simulink model "different_inverter_controls_BPS"  (R2024b)
settings: Solver=ode4  StartTime=0.0  StopTime=5  FixedStep=Ts  RelTol=1e-3
InitFcn:
  | %mode_of_operation=1;
  | %BESS_control_mode=1;
  | %Gen_Q_Control =1;
  | 
  | %Exciter_init;
  | 
  | %Exciter_init
  | Xq=0.474;
  | %%====================================================
  | % ST6C Exciter Parameters
  | 
  | KPA=30;
  | KIA=59.91;
  | KFF=1;
  | KM=1;
  | KLR=22.47;
  | KCL=1.04;
  | VAMAX=7.05;
  | VAMIN=-6.11;
  | VRMAX=7.05;
  | VRMIN=-6.11;
  | ILR=5.02;
  | KG=1;
  | TG=0.024;
  | TA=0.01;
  | VBMAX=999;
  | VMMAX=7.05;
  | VMMIN=-6.11;
  | KI=0;
  | Kp=1;
  | Kc=0;
  | Vt0=0;
  | VAAMAX=VAMAX;
  | %%========================================================
  | % UEL2C parameters
  | 
  | TUQ=.005;
  | TUP=0.050;
  | TUV=0.2;
  | TQREF=0;
  | Tadj=0;
  | K1=0;
  | K2=2;
  | VBIAS=1;
  | KFB=0;
  | TUL=0;
  | VUImax=1;
  | VUImin=-1;
  | VUELmax1=1;
  | VUELmax2=1;
  | VUELmin1=-1;
  | VUELmin2=-1;
  | KUF=0;
  | KUL=0.24;
  | KUI=0.001;
  | TU1=0;TU2=0;TU3=0;TU4=0;
  | KFIX=1;
  | VF=0;
  | VFB=0;
  | %%===========================================================
  | ... (+60 lines)
values from neighbouring files (symbols this model uses):
  inv1 = struct    [multiInverterParams.m]
  kp_sync = KQ_p/10    (= 0.04)    [multiInverterParams.m]
  Vdc = 1000    [multiInverterParams.m]
  Vpp = 480    [multiInverterParams.m]
undefined symbols (not defined in the file or in its folder): D1, Delta, DiscIntNeverNeededParam, Ion, Lithium, sigbuilder_block, sps
libraries: slpidlib x34, spsThreePhaseVIMeasurementLib x31, spsThreePhaseSeriesRLCBranchLib x23, spsabctodq0Lib x22, spsPower3phInstantaneousLib x22, spsThreePhaseTransformerTwoWindingsLib x16, spsSeriesRLCBranchLib x16, spsThreePhaseSeriesRLCLoadLib x14, simulink x12, spsPLL3phLib x11, spsGroundLib x9, powerlib_extras x8
(part 2 of 9)

== system different_inverter_controls_BPS/IBR-GFM Synchro-inverter/Inverter ==
  " Reference " : Subsystem
  "            VDC1" : spsDCVoltageSourceLib/DC Voltage Source  Amplitude=Vdc  Measurements=None
  Bus Selector : BusSelector  OutputSignals=Vabc,Iabc
  DC Link : Subsystem
  From1 : From  Commented=on  GotoTag=m_batt
  From2 : From  Commented=on  GotoTag=m_inv
  Goto Tag Visibility : GotoTagVisibility  GotoTag=PLL_Freq
  Grid Inverter : Subsystem
  Inverter Control : Subsystem
  Measures : Subsystem  Commented=on
  Power Controller : Subsystem  SystemSampleTime=Ts
  Rate Transition2 : RateTransition  OutPortSampleTime=Ts_Control
  Scope : Scope
  Scope1 : Scope
  Voltage Measurement : spsVoltageMeasurementLib/Voltage Measurement  PhasorSimulation=off  OutputType=Complex  PSBequivalent=0
  A : PMIOPort  Side=Right
  B : PMIOPort  Port=2  Side=Right
  C : PMIOPort  Port=3  Side=Right
  m : Outport  VectorParamsAs1DForOutWhenUnconnected=off
  tag scope: Uref=global
  wires:
  [V_inv_mag] -> Inverter Control/5(V_inv_mag)
  [V_inv_mag] -> Power Controller/5(V_inv_mag)
  Voltage Measurement/1 -> Scope1/1
  Power Controller/2(Vdref) -> Inverter Control/4(Vdref)
  [BESS_PQf_ref] -> Power Controller/2(PQref_f)
  Rate Transition2/1 -> Bus Selector/1, Power Controller/1(m_PQ)
  Inverter Control/1(Uref) -> [Uref], Scope/1, Grid Inverter/1(Uref)
  Bus Selector/1 -> Inverter Control/1(Vabc_prim)  "<Vabc>"
  Bus Selector/2 -> Inverter Control/2(Iabc_prim)  "<Iabc>"
  Grid Inverter/1(m) -> [m_inv]
  From2/1 -> Measures/1(Grid)
  From1/1 -> Measures/2(Battery)
  Measures/1(m) -> m/1
  [m_inv] -> Rate Transition2/1
  Power Controller/1(theta) -> Inverter Control/3(theta)
  [theta_wt] -> Power Controller/3(Input)
  [f_system] -> Power Controller/4(fsys)
  connections:
  "            VDC1"/RConn1 -- DC Link/LConn1
  DC Link/LConn2 -- "            VDC1"/LConn1
  DC Link/RConn3 -- Voltage Measurement/LConn2 -- Grid Inverter/LConn3
  A/RConn1 -- Grid Inverter/RConn1
  B/RConn1 -- Grid Inverter/RConn2
  C/RConn1 -- Grid Inverter/RConn3
  DC Link/RConn1 -- Voltage Measurement/LConn1 -- Grid Inverter/LConn1
  DC Link/RConn2 -- Grid Inverter/LConn2

== system different_inverter_controls_BPS/IBR-GFM Power Synchronization/Inverter ==
  " Reference " : Subsystem
  "            VDC1" : spsDCVoltageSourceLib/DC Voltage Source  Amplitude=Vdc  Measurements=None
  Battery2 : spsBatteryLib/Battery  Commented=on  BatType=Lithium-Ion  NomV=1000  NomQ=Bcap  SOC=100  Batt_Tr=1  PresetModel=on  MaxQ=110000  MinV=750  FullV=1163.9871  Dis_rate=47826.087  R=9.0909e-05  Normal_OP=99478.2609  expZone="[1080.3859      5404.3478]"
  Bus Selector : BusSelector  OutputSignals=Vabc,Iabc
  DC Link : Subsystem
  From1 : From  Commented=on  GotoTag=m_batt
  From2 : From  Commented=on  GotoTag=m_inv
  Goto Tag Visibility : GotoTagVisibility  GotoTag=PLL_Freq
  Goto3 : Goto  Commented=on  GotoTag=m_batt
  Grid Inverter : Subsystem
  Inverter Control : Subsystem
  Measures : Subsystem  Commented=on
  Power Controller : Subsystem  SystemSampleTime=Ts
  Rate Transition2 : RateTransition  OutPortSampleTime=Ts_Control
  Scope : Scope
  Scope1 : Scope
  Voltage Measurement : spsVoltageMeasurementLib/Voltage Measurement  PhasorSimulation=off  OutputType=Complex  PSBequivalent=0
  A : PMIOPort  Side=Right
  B : PMIOPort  Port=2  Side=Right
  C : PMIOPort  Port=3  Side=Right
  m : Outport  VectorParamsAs1DForOutWhenUnconnected=off
  tag scope: Uref=global
  wires:
  [V_inv_mag] -> Inverter Control/5(V_inv_mag)
  [V_inv_mag] -> Power Controller/5(V_inv_mag)
  Voltage Measurement/1 -> Scope1/1
  Battery2/1 -> Goto3/1
  Power Controller/2(Vdref) -> Inverter Control/4(Vdref)
  [BESS_PQf_ref] -> Power Controller/2(PQref_f)
  Rate Transition2/1 -> Bus Selector/1, Power Controller/1(m_PQ)
  Inverter Control/1(Uref) -> [Uref], Scope/1, Grid Inverter/1(Uref)
  Bus Selector/1 -> Inverter Control/1(Vabc_prim)  "<Vabc>"
  Bus Selector/2 -> Inverter Control/2(Iabc_prim)  "<Iabc>"
  Grid Inverter/1(m) -> [m_inv]
  From2/1 -> Measures/1(Grid)
  From1/1 -> Measures/2(Battery)
  Measures/1(m) -> m/1
  [m_inv] -> Rate Transition2/1
  Power Controller/1(theta) -> Inverter Control/3(theta)
  [theta_wt] -> Power Controller/3(Input)
  [f_system] -> Power Controller/4(fsys)
  connections:
  "            VDC1"/RConn1 -- DC Link/LConn1
  DC Link/LConn2 -- "            VDC1"/LConn1
  DC Link/RConn3 -- Voltage Measurement/LConn2 -- Grid Inverter/LConn3
  A/RConn1 -- Grid Inverter/RConn1
  B/RConn1 -- Grid Inverter/RConn2
  C/RConn1 -- Grid Inverter/RConn3
  DC Link/RConn1 -- Voltage Measurement/LConn1 -- Grid Inverter/LConn1
  DC Link/RConn2 -- Grid Inverter/LConn2

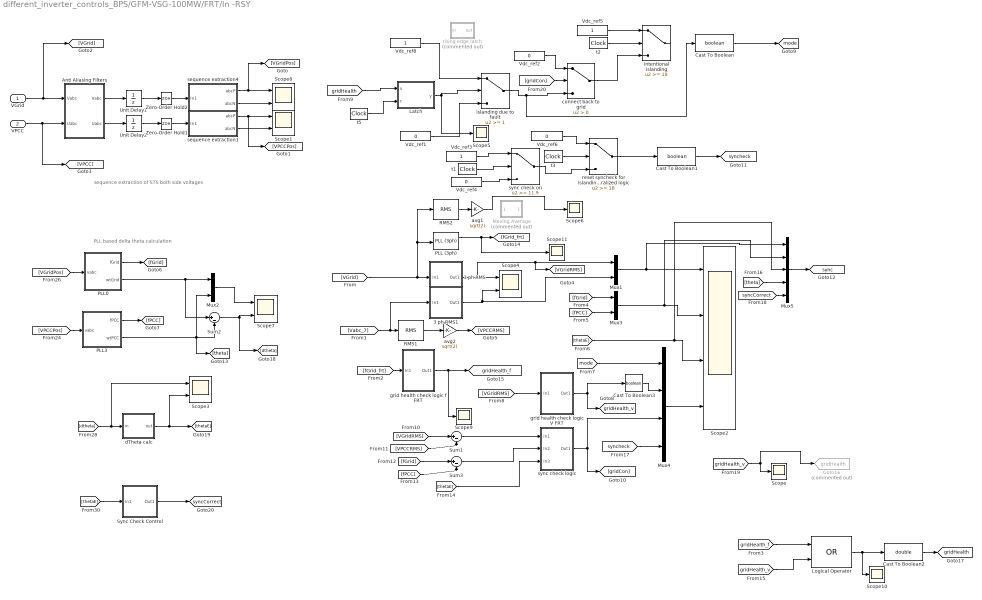
== system different_inverter_controls_BPS/GFM-VSG-100MW/FRT/In -RSY ==
  note: PLL based delta theta calculation
  note: sequence extraction of STS both side voltages
  VGrid : Inport
  VPCC : Inport  Port=2
  3 ph RMS : Subsystem
  3 ph RMS1 : Subsystem
  Anti Aliasing Filters : Subsystem  mask(Anti-aliasing (2nd order lowpass)){Fc=300, Ts=Ts}
      mask prompts: Fc "Cut-off frequency (Hz):"; Ts "Sample time:"
  Cast To Boolean : DataTypeConversion  OutDataTypeStr=boolean  SaturateOnIntegerOverflow=off  RndMeth=Floor
  Cast To Boolean1 : DataTypeConversion  OutDataTypeStr=boolean  SaturateOnIntegerOverflow=off  RndMeth=Floor
  Cast To Boolean2 : DataTypeConversion  OutDataTypeStr=double  SaturateOnIntegerOverflow=off  RndMeth=Floor
  Cast To Boolean3 : DataTypeConversion  OutDataTypeStr=boolean  SaturateOnIntegerOverflow=off  RndMeth=Floor
  Goto16 : Goto  Commented=on  GotoTag=gridHealth  TagVisibility=global
  Latch : MATLAB Function  TreatAsAtomicUnit=on
  Logical Operator : Logic  Operator=OR  AllPortsSameDT=off  OutDataTypeStr=boolean
  Moving Average : Subsystem  Description=Replaced Block  Commented=on  InitFcn=error('This block was designed with a newer version of Simulink. Unfortunately, your Simulink version does not support these features.')  mask(Replaced Block){}
      mask help: This block has been replaced with an empty subsystem because it used functionality that is unavailable in Simulink R2021a.
      mask Display: fprintf('Replaced: %s\n','Moving Statistics with Overlap Length not equal to Window Length - 1 (supported from R2022b).')
  Mux1 : Mux  Inputs=2
  Mux2 : Mux  Inputs=2
  Mux3 : Mux  Inputs=2
  Mux4 : Mux
  Mux5 : Mux  Inputs=5
  PLL (3ph) : spsPLL3phLib/PLL (3ph)  Fmin=45  Par_Init=[0, 60]  ParK=[180, 3200, 1]  TcD=1e-4  MaxRateChangeFreq=12  FilterCutOffFreq=25  Ts=0  AGC=on
  PLL0 : Subsystem
  PLL3 : Subsystem
  RMS1 : spsRMSLib/RMS  TrueRMS=on  Freq=f  RMSInit=1  Ts=0
  RMS2 : spsRMSLib/RMS  TrueRMS=on  Freq=f  RMSInit=1  Ts=0
  Scope{,5..6,9..11} (6 alike) : Scope
  Scope{1,3..4,7..8} (5 alike) : Scope  NumInputPorts=2
  Scope2 : Scope  NumInputPorts=4
  Sum1 : Sum  Inputs=|+-
  Sum2 : Sum  Inputs=|+-
  Sum3 : Sum  Inputs=|+-
  Sync Check Control : Subsystem
  Unit Delay1 : UnitDelay  InitialCondition=1  SampleTime=Ts  HasFrameUpgradeWarning=on
  Unit Delay2 : UnitDelay  InitialCondition=1  SampleTime=Ts  HasFrameUpgradeWarning=on
  Vdc_ref{1..2,4,6} (4 alike) : Constant  Value=0  SampleTime=Ts
  Vdc_ref3 : Constant  SampleTime=Ts
  Vdc_ref5 : Constant  SampleTime=Ts
  Vdc_ref8 : Constant  SampleTime=Ts
  Zero-Order Hold1 : ZeroOrderHold  SampleTime=Ts_Control
  Zero-Order Hold2 : ZeroOrderHold  SampleTime=Ts_Control
  avg1 : Gain  Gain=sqrt(2)
  avg2 : Gain  Gain=sqrt(2)
  connect back to grid : Switch  Criteria=u2 > Threshold  SaturateOnIntegerOverflow=off  InputSameDT=off
  dTheta calc : MATLAB Function  TreatAsAtomicUnit=on
  grid health check logic V FRT : Subsystem
  grid health check logic f FRT : Subsystem
  intentional islanding : Switch  Threshold=18  SaturateOnIntegerOverflow=off  InputSameDT=off
  islanding due to fault : Switch  Threshold=1  SaturateOnIntegerOverflow=off  InputSameDT=off
  reset syncheck for islanding not a generalized logic : Switch  Threshold=18  SaturateOnIntegerOverflow=off  InputSameDT=off
  rising edge latch : MATLAB Function  Commented=on  TreatAsAtomicUnit=on
  sequence extraction1 : Subsystem
  sequence extraction4 : Subsystem
  sync check logic : Subsystem
  sync check on : Switch  Threshold=11.9  SaturateOnIntegerOverflow=off  InputSameDT=off
  t{1..3,5} (4 alike) : DigitalClock  SampleTime=Ts
  tag scope: gridHealth=global, gridHealth_f=global, gridHealth_v=global, mode=global, sync=global, syncCorrect=global, syncheck=global
  wires:
  Vdc_ref1/1 -> islanding due to fault/3
  islanding due to fault/1 -> Cast To Boolean/1, connect back to grid/3
  VGrid/1 -> [VGrid], Anti Aliasing Filters/1(Vabc)
  VPCC/1 -> [VPCC], Anti Aliasing Filters/2(Uabc)
  [dtheta] -> Scope3/1, dTheta calc/1(in)
  [VPCCPos] -> PLL3/1(vabc)
  Mux2/1 -> Scope7/1
  dTheta calc/1(out) -> Scope3/2, [thetaE]
  PLL3/2(wtPCC) -> [theta], Mux2/2, Sum2/2
  Sum2/1 -> Scope7/2, [dtheta]
  Unit Delay1/1 -> Zero-Order Hold2/1
  Anti Aliasing Filters/1(" Vabc") -> Unit Delay1/1
  Unit Delay2/1 -> Zero-Order Hold1/1
  Anti Aliasing Filters/2(" Uabc") -> Unit Delay2/1
  sequence extraction4/2(abcN) -> Scope8/2
  sequence extraction4/1(abcP) -> [VGridPos], Scope8/1
  Zero-Order Hold2/1 -> sequence extraction4/1(In1)
  Zero-Order Hold1/1 -> sequence extraction1/1(In1)
  sequence extraction1/1(abcP) -> [VPCCPos], Scope1/1
  sequence extraction1/2(abcN) -> Scope1/2
  [VGridPos] -> PLL0/1(vabc)
  PLL0/2(wtGrid) -> Sum2/1, Mux2/1
  [Vabc_7] -> 3 ph RMS1/1(In1), RMS1/1
  PLL0/1(fGrid) -> [fGrid]
  PLL3/1(fPCC) -> [fPCC]
  [fGrid] -> Mux3/1
  [fPCC] -> Mux3/2
  Mux1/1 -> Mux5/1, Scope2/1
  Mux3/1 -> Mux5/2, Scope2/2
  [thetaE] -> Mux5/3, Scope2/3
  [VGridRMS] -> grid health check logic V FRT/1(In1)
  grid health check logic V FRT/1(Out1) -> Cast To Boolean3/1, [gridHealth_v]
  [mode] -> Mux4/1
  Mux4/1 -> Scope2/4
  [VGridRMS] -> Sum1/1
  [VPCCRMS] -> Sum1/2
  [fGrid] -> Sum3/1
  [fPCC] -> Sum3/2
  Sum1/1 -> sync check logic/1(In1)
  Sum3/1 -> sync check logic/2(In2)
  [thetaE] -> sync check logic/3(In3)
  sync check logic/1(Out1) -> [gridCon], Mux4/3
  t1/1 -> sync check on/2
  Vdc_ref3/1 -> sync check on/1
  Vdc_ref4/1 -> sync check on/3
  Cast To Boolean3/1 -> Mux4/2
  Cast To Boolean1/1 -> [syncheck]
  [syncheck] -> Mux4/4
  Vdc_ref5/1 -> intentional islanding/1
  t2/1 -> intentional islanding/2
  sync check on/1 -> reset syncheck for islanding not a generalized logic/3
  reset syncheck for islanding not a generalized logic/1 -> Cast To Boolean1/1
  Vdc_ref6/1 -> reset syncheck for islanding not a generalized logic/1
  t3/1 -> reset syncheck for islanding not a generalized logic/2
  Sync Check Control/1(Out1) -> [syncCorrect]
  [thetaE] -> Sync Check Control/1(In1)
  RMS2/1 -> avg1/1
  [VGrid] -> PLL (3ph)/1, RMS2/1, 3 ph RMS/1(In1)
  avg2/1 -> [VPCCRMS]
  RMS1/1 -> avg2/1
  Mux5/1 -> [sync]
  [theta] -> Mux5/4
  [syncCorrect] -> Mux5/5
  connect back to grid/1 -> intentional islanding/3
  3 ph RMS/1(Out1) -> [VGridRMS], Mux1/1, Scope4/1
  3 ph RMS1/1(Out1) -> Mux1/2, Scope4/2
  PLL (3ph)/1 -> Scope11/1, [fGrid_frt]
  grid health check logic f FRT/1(Out1) -> Scope9/1, [gridHealth_f]
  [fGrid_frt] -> grid health check logic f FRT/1(In1)
  [gridHealth_v] -> Goto16/1, Scope/1
  Cast To Boolean/1 -> [mode]
  [gridHealth] -> Latch/1(u)
  Vdc_ref8/1 -> islanding due to fault/1
  Latch/1(y) -> islanding due to fault/2, Scope5/1
  t5/1 -> Latch/2(c)
  [gridCon] -> connect back to grid/2
  Vdc_ref2/1 -> connect back to grid/1
  [gridHealth_f] -> Logical Operator/1
  [gridHealth_v] -> Logical Operator/2
  Logical Operator/1 -> Cast To Boolean2/1, Scope10/1
  Cast To Boolean2/1 -> [gridHealth]
  avg1/1 -> Scope6/1

== system different_inverter_controls_BPS/GFM-VSG-100MW/IBR-GFM VSG/Inverter ==
  "            VDC1" : spsDCVoltageSourceLib/DC Voltage Source  Amplitude=Vdc  Measurements=None
  "BESS Reference " : Subsystem
  Bus Selector : BusSelector  OutputSignals=Vabc,Iabc
  DC Link : Subsystem
  From1 : From  Commented=on  GotoTag=m_batt
  From2 : From  Commented=on  GotoTag=m_inv
  Goto Tag Visibility : GotoTagVisibility  GotoTag=PLL_Freq
  Grid Inverter : Subsystem
  Inverter Control : Subsystem
  Measures : Subsystem  Commented=on
  Power Controller : Subsystem  SystemSampleTime=Ts
  Rate Transition2 : RateTransition  OutPortSampleTime=Ts_Control
  Scope : Scope
  Scope1 : Scope
  Voltage Measurement : spsVoltageMeasurementLib/Voltage Measurement  PhasorSimulation=off  OutputType=Complex  PSBequivalent=0
  A : PMIOPort  Side=Right
  B : PMIOPort  Port=2  Side=Right
  C : PMIOPort  Port=3  Side=Right
  m : Outport  VectorParamsAs1DForOutWhenUnconnected=off
  tag scope: Uref=global
  wires:
  Power Controller/1(theta) -> Inverter Control/3(theta)
  [m_inv] -> Rate Transition2/1
  Measures/1(m) -> m/1
  From1/1 -> Measures/2(Battery)
  From2/1 -> Measures/1(Grid)
  Grid Inverter/1(m) -> [m_inv]
  Bus Selector/2 -> Inverter Control/2(Iabc_prim)  "<Iabc>"
  Bus Selector/1 -> Inverter Control/1(Vabc_prim)  "<Vabc>"
  Inverter Control/1(Uref) -> Grid Inverter/1(Uref), Scope/1, [Uref]
  Rate Transition2/1 -> Power Controller/1(m_PQ), Bus Selector/1
  [BESS_PQf_ref] -> Power Controller/2(PQref_f)
  Power Controller/2(Vdref) -> Inverter Control/4(Vdref)
  Voltage Measurement/1 -> Scope1/1
  [V_inv_mag] -> Power Controller/3(V_inv_mag)
  [V_inv_mag] -> Inverter Control/5(V_inv_mag)
  connections:
  DC Link/RConn2 -- Grid Inverter/LConn2
  Grid Inverter/LConn1 -- Voltage Measurement/LConn1 -- DC Link/RConn1
  C/RConn1 -- Grid Inverter/RConn3
  B/RConn1 -- Grid Inverter/RConn2
  A/RConn1 -- Grid Inverter/RConn1
  Grid Inverter/LConn3 -- Voltage Measurement/LConn2 -- DC Link/RConn3
  DC Link/LConn2 -- "            VDC1"/LConn1
  "            VDC1"/RConn1 -- DC Link/LConn1

== system different_inverter_controls_BPS/GT-swing/Gen-a/Synchronous Machine G2 50 MVA 16.5 kV ==
  note: Reactive Power
  note: Field Current
  note: Stator Current
  note: Stator Voltage
  note: Active Power
  note: Rotor Speed
  note: Selected (Combined)
      | Synchronous Machine
      | Measurement Outputs
  note: Synchronous
      | Machine
      | - Phase A
      | - Phase B
      | - Phase C
  note: SM Measurement Signal
  note: Rotor Speed Reference
  note: Rotor Speed
  note: Stator Current
  note: Reactive Power
  note: Stator Voltage
  note: Voltage Reference
  note: Field Current
  note: Active Power
  note: Field Voltage (Vf)
  note: Mechanical
      | Power (Pm)
  wref (pu) : Inport
  Vref (pu) : Inport  Port=2
  Generator Measurements (Output) : Subsystem
  Governor model with Droop : Subsystem
  Ground7 : Ground
  ST6C EXCITER-1 : Subsystem
  Synchronous Machine : spsSynchronousMachinepuStandardLib/Synchronous Machine pu Standard  PresetModel=No  MechanicalLoad=Mechanical power Pm  ShowDetailedParameters=on  RotorType=Salient-pole  Units=per unit standard parameters  MeasurementBus=off  NominalParameters="[ Pn  Vn   f ]"  Reactances1=[ 31 32 33 34 35 36 37 ]  Reactances2=[ 1.305, 0.296, 0.252, 0.474, 0.243, 0.18 ]  dAxisTimeConstants=Short-circuit  qAxisTimeConstants=Open-circuit  TimeConstants1=[]  TimeConstants2=[]  TimeConstants3=[]  TimeConstants4=[]  TimeConstants5=[ 1.01, 0.053, 0.1 ]  TimeConstants6=[]  TimeConstants7=[]  TimeConstants8=[]  StatorResistance=2.8544e-3  Mechanical=[H2 0 2]  PolePairs=2  InitialConditions=[0 -83.8079 0.361964 0.361964 0.361964 -44.5111 -164.511 75.4889 1.36037]  SetSaturation=off  Saturation=[0.6404,0.7127,0.8441,0.9214,0.9956,1.082,1.19,1.316,1.457;0.7,0.7698,0.8872,0.9466,0.9969,1.046,1.1,1.151,1.201]  LoadFlowParameters=[1 150000000 0 0]  TsPowergui=0  TsBlock=-1  IterativeModel=Trapezoidal non iterative  IterativeDiscreteModel=Trapezoidal non iterative  BusType=swing  Pref=100000000  Qref=0  Qmin=-50000000  Qmax=50000000  PLF=0  QLF=0
  A : PMIOPort  Side=Right
  B : PMIOPort  Port=2  Side=Right
  C : PMIOPort  Port=3  Side=Right
  sms : Outport  VectorParamsAs1DForOutWhenUnconnected=off
  wires:
  Vref (pu)/1 -> ST6C EXCITER-1/1(Vref)
  Governor model with Droop/1(Pmec (pu)) -> Synchronous Machine/1
  Ground7/1 -> ST6C EXCITER-1/5(Vstab)
  [QT2nds] -> ST6C EXCITER-1/6(QT)
  [It2nds] -> ST6C EXCITER-1/3(It)
  [PT2nds] -> ST6C EXCITER-1/7(PT)
  wref (pu)/1 -> Governor model with Droop/1(wref (pu)1)
  ST6C EXCITER-1/1(Efd) -> Synchronous Machine/2, [Efd2nds]
  Generator Measurements (Output)/2(wm) -> [wms]
  Generator Measurements (Output)/4(Ifd) -> [Ifd2nds]
  Generator Measurements (Output)/5(It) -> [It2nds]
  Generator Measurements (Output)/1(sm) -> sms/1
  Generator Measurements (Output)/7(QT) -> [QT2nds]
  Generator Measurements (Output)/6(PT) -> [PT2nds]
  Generator Measurements (Output)/3(Vt) -> [Vt2nds]
  Synchronous Machine/1 -> Generator Measurements (Output)/1(m)
  [wms] -> Governor model with Droop/2(w (pu))
  [Vt2nds] -> ST6C EXCITER-1/2(Vt)
  [Ifd2nds] -> ST6C EXCITER-1/4(Ifd)
  connections:
  B/RConn1 -- Synchronous Machine/RConn2
  C/RConn1 -- Synchronous Machine/RConn3
  A/RConn1 -- Synchronous Machine/RConn1

== system different_inverter_controls_BPS/IBR GFL-SH/BESS/BESS Reference  ==
  Clock : Clock  Commented=on
  Constant1 : Constant  Value=0  SampleTime=Ts_Control
  Digital Clock : DigitalClock  SampleTime=Ts_Control
  If : If  IfExpression=u1>=0
  If Action Subsystem : Subsystem  TreatAsAtomicUnit=on
  If Action Subsystem1 : Subsystem  TreatAsAtomicUnit=on
  Merge : Merge
  Mux3 : Mux  Inputs=2
  Pref : Subsystem
  Qref : Subsystem
  Scope : Scope
  tag scope: BESS_PQf_ref=global
  wires:
  Merge/1 -> Mux3/1
  Qref/1(Out1) -> Mux3/2
  Constant1/1 -> If Action Subsystem1/1(In1)
  If Action Subsystem/1(Out1) -> Merge/1
  If/1 -> If Action Subsystem/Action
  Pref/1(Out1) -> If Action Subsystem/1(In1)
  If/2 -> If Action Subsystem1/Action
  If Action Subsystem1/1(Out1) -> Merge/2
  Mux3/1 -> [BESS_PQf_ref], Scope/1
  Digital Clock/1 -> If/1

== system different_inverter_controls_BPS/IBR GFL-SH/BESS/DC Link ==
  C1 : spsSeriesRLCBranchLib/Series RLC Branch  LConnTagsString=__new0  RConnTagsString=__new0  BranchType=C  Resistance=1.0  Inductance=1.0  SetiL0=off  InitialCurrent=0  Capacitance=Clink  Setx0=on  InitialVoltage=Vnom_dc/2  Measurements=None
  C2 : spsSeriesRLCBranchLib/Series RLC Branch  LConnTagsString=__new0  RConnTagsString=__new0  BranchType=C  Resistance=1e5  Inductance=1.0  SetiL0=off  InitialCurrent=0  Capacitance=Clink  Setx0=on  InitialVoltage=Vnom_dc/2  Measurements=None
  PV+ : PMIOPort  Side=Left
  PV-- : PMIOPort  Port=2  Side=Left
  Inv+ : PMIOPort  Port=3  Side=Right
  N : PMIOPort  Port=4  Side=Right
  Inv-- : PMIOPort  Port=5  Side=Right
  connections:
  Inv--/RConn1 -- PV--/RConn1 -- C2/RConn1
  C1/RConn1 -- N/RConn1 -- C2/LConn1
  Inv+/RConn1 -- PV+/RConn1 -- C1/LConn1

== system different_inverter_controls_BPS/IBR GFL-SH/BESS/Grid Inverter ==
  note: Harmonic Filter
  Uref : Inport
  10 kvar : spsThreePhaseSeriesRLCLoadLib/Three-Phase Series RLC Load  LConnTagsString=A|B|C  Configuration=Delta  NominalVoltage=Vnom_sec  Vabc=[1e3 1e3 1e3]  Vabcp=[1e3 1e3 1e3]  NominalFrequency=Fnom  UnbalancedPower=off  ActivePower=Pc  InductivePower=0  CapacitivePower=Qc  Pabc=[10e3 9e3 11e3]  QLabc=[100 90 110]  QCabc=[100 90 110]  Pabcp=[10e3 9e3 11e3]  QLabcp=[100 90 110]  QCabcp=[100 90 110]  Measurements=None  LoadType=constant Z
  B1 : spsThreePhaseVIMeasurementLib/Three-Phase V-I Measurement  VoltageMeasurement=phase-to-ground  SetLabelV=off  LabelV=Vabc_B1  Vpu=off  VpuLL=off  CurrentMeasurement=yes  SetLabelI=off  LabelI=Iabc_B1  Ipu=off  Pbase=100e6  Vbase=500e3  OutputType=Magnitude  PhasorSimulation=off  PSBequivalent=0
  Bus Creator : BusCreator  Inputs=2
  Ground : Ground
  L : spsThreePhaseSeriesRLCBranchLib/Three-Phase Series RLC Branch  LConnTagsString=A|B|C  RConnTagsString=A|B|C  BranchType=RL  Resistance=Rchoke*Zbase  Inductance=Lchoke*Zbase/(2*pi*Fnom)  Capacitance=inf  Measurements=None
  Scope : Scope
  Scope1 : Scope
  Three-Level NPC Converter : spsThreeLevelNPCConverterLib/Three-Level NPC Converter  ModelType=Average model (Uref-controlled)  Ron=1e-3  Rs=1e6  Cs=inf  Vforward=[0,0]  Ron_Diode=1e-3  Rs_Diode=1e6  Cs_Diode=inf  Vf_Diode=1e-3  Rs_CurrentSource=inf  Ron_ACsource=1e-3
  XFR : spsThreePhaseTransformerTwoWindingsLib/Three-Phase Transformer (Two Windings)  Winding1Connection=Delta (D1)  Winding2Connection=Delta (D1)  CoreType=Three single-phase transformers  SetSaturation=off  Hysteresis=off  DataFile='hysteresis'  SetInitialFlux=off  Measurements=None  UNITS=pu  NominalPower=[100e6, f ]  Winding1="[Vnom_prim,  1e-6, 0.0586 ]"  Winding2="[ Vnom_sec,  1e-6, 0.0586 ]"  Rm=500  Lm=500  L0=0.5  Saturation=[ 0,0 ; 0.0024,1.2 ; 1.0,1.52 ]  InitialFluxes=[ 0.8 , -0.8 , 0.7 ]  BreakLoop=off  DiscreteSolver=Trapezoidal iterative  DataType=off  TransfoNumber=1
  Inv+ : PMIOPort  Side=Left
  N : PMIOPort  Port=2  Side=Left
  Inv-- : PMIOPort  Port=3  Side=Left
  A : PMIOPort  Port=4  Side=Right
  B : PMIOPort  Port=5  Side=Right
  C : PMIOPort  Port=6  Side=Right
  m : Outport  VectorParamsAs1DForOutWhenUnconnected=off
  wires:
  Uref/1 -> Three-Level NPC Converter/1
  B1/1 -> Scope/1, Bus Creator/1  "Vabc"
  B1/2 -> Scope1/1, Bus Creator/2  "Iabc"
  Bus Creator/1 -> m/1
  Ground/1 -> Three-Level NPC Converter/2
  connections:
  B1/RConn3 -- C/RConn1
  B1/RConn2 -- B/RConn1
  B1/RConn1 -- A/RConn1
  10 kvar/LConn1 -- XFR/RConn1 -- L/RConn1
  Three-Level NPC Converter/RConn1 -- Inv+/RConn1
  Three-Level NPC Converter/RConn3 -- Inv--/RConn1
  L/RConn3 -- XFR/RConn3 -- 10 kvar/LConn3
  L/RConn2 -- XFR/RConn2 -- 10 kvar/LConn2
  XFR/LConn3 -- B1/LConn3
  XFR/LConn2 -- B1/LConn2
  XFR/LConn1 -- B1/LConn1
  Three-Level NPC Converter/LConn1 -- L/LConn1
  Three-Level NPC Converter/LConn2 -- L/LConn2
  Three-Level NPC Converter/LConn3 -- L/LConn3
  N/RConn1 -- Three-Level NPC Converter/RConn2

== system different_inverter_controls_BPS/IBR GFL-SH/BESS/Inverter Control ==
  Vabc_prim : Inport  PortDimensions=3
  Iabc_prim : Inport  Port=2  PortDimensions=3
  Idq_ref : Inport  Port=3
  Current Control : Subsystem  TreatAsAtomicUnit=on
  Demux : Demux  Outputs=2
  Overmodulation : spsOvermodulationLib/Overmodulation  Commented=through  OverModType=Flat top
  Scope : Scope  NumInputPorts=2
  Unit Delay : UnitDelay  SampleTime=Ts_Control  HasFrameUpgradeWarning=on
  Voltage Loop : Subsystem
  current limiter : Subsystem  mask{limMax=clMax, limMin=clMin}
      mask prompts: limMax "Max current limit (pu)"; limMin "Min current limit (pu)"
  Uref : Outport  VectorParamsAs1DForOutWhenUnconnected=off
  wires:
  [IdIqref] -> Current Control/4(IdIq_ref)
  [idiqPRef] -> Scope/2
  [wt] -> Current Control/1(wt)
  Idq_ref/1 -> [IdIqref]
  Voltage Loop/1(wt) -> [wt]
  Demux/2 -> [Vq_meas]
  Demux/1 -> [Vd_meas]
  Vabc_prim/1 -> Voltage Loop/1(Vabc_prim)
  [idiqPRefL] -> Current Control/3(IdIq_meas)
  Voltage Loop/3(IdIq_prim) -> [idiqPRef]
  [idiqPRef] -> current limiter/1(idiqPref)
  current limiter/1(idiqPRefL) -> Scope/1, [idiqPRefL]
  Unit Delay/1 -> Overmodulation/1
  Overmodulation/1 -> Uref/1
  Current Control/1(Uabc) -> Unit Delay/1
  Voltage Loop/2(VdVq_prim) -> Demux/1, Current Control/2(VdVq_meas)
  Iabc_prim/1 -> Voltage Loop/2(Iabc_prim)

== system different_inverter_controls_BPS/IBR GFL-SH/BESS/Measures ==
  Grid : Inport
  Battery : Inport  Port=2
  Bus Creator : BusCreator  Inputs=2
  Bus Creator1 : BusCreator  Inputs=4
  Bus Selector2 : BusSelector  OutputSignals=Vabc,Iabc
  "Power (3ph, Instantaneous)" : spsPower3phInstantaneousLib/Power (3ph, Instantaneous)
  Scope : Scope
  m : Outport  VectorParamsAs1DForOutWhenUnconnected=off
  wires:
  Bus Creator1/1 -> Bus Creator/1  "Grid"
  "Power (3ph, Instantaneous)"/2 -> Bus Creator1/4  "Q"
  Grid/1 -> Bus Selector2/1
  Battery/1 -> Bus Creator/2  "Battery"
  Bus Creator/1 -> m/1
  "Power (3ph, Instantaneous)"/1 -> Scope/1, Bus Creator1/3  "P"
  Bus Selector2/2 -> Bus Creator1/2, "Power (3ph, Instantaneous)"/2  "<Iabc>"
  Bus Selector2/1 -> Bus Creator1/1, "Power (3ph, Instantaneous)"/1  "<Vabc>"

== system different_inverter_controls_BPS/IBR GFL-SH/BESS/Power Control Loop ==
  m_PQ : Inport
  PQref_f : Inport  Port=2
  Compute PQ : Subsystem
  "P,Q Control " : Subsystem  TreatAsAtomicUnit=on
  to PU : Gain  Gain=1/Pnom
  Idq_ref : Outport  VectorParamsAs1DForOutWhenUnconnected=off
  wires:
  to PU/1 -> "P,Q Control "/1(PQref)
  m_PQ/1 -> Compute PQ/1(m)
  Compute PQ/1(PQm) -> "P,Q Control "/2(m)
  "P,Q Control "/1(Idq_ref) -> Idq_ref/1
  PQref_f/1 -> to PU/1

== system different_inverter_controls_BPS/IBR GFL-SH/IBR/ Reference  ==
  Mux3 : Mux  Inputs=2
  Pref : Subsystem
  Qref : Subsystem
  Scope : Scope
  tag scope: PQf_ref=global, Pref_plot=global, Qref_plot=global
  wires:
  Qref/1(Out1) -> [Qref_plot], Mux3/2
  Mux3/1 -> [PQf_ref], Scope/1
  Pref/1(Out1) -> [Pref_plot], Mux3/1

== system different_inverter_controls_BPS/IBR GFL-SH/IBR/DC Link ==
  C1 : spsSeriesRLCBranchLib/Series RLC Branch  LConnTagsString=__new0  RConnTagsString=__new0  BranchType=RC  Resistance=1.0  Inductance=1.0  SetiL0=off  InitialCurrent=0  Capacitance=Clink  Setx0=on  InitialVoltage=Vnom_dc/2  Measurements=None
  C2 : spsSeriesRLCBranchLib/Series RLC Branch  LConnTagsString=__new0  RConnTagsString=__new0  BranchType=RC  Resistance=1e5  Inductance=1.0  SetiL0=off  InitialCurrent=0  Capacitance=Clink  Setx0=on  InitialVoltage=Vnom_dc/2  Measurements=None
  PV+ : PMIOPort  Side=Left
  PV-- : PMIOPort  Port=2  Side=Left
  Inv+ : PMIOPort  Port=3  Side=Right
  N : PMIOPort  Port=4  Side=Right
  Inv-- : PMIOPort  Port=5  Side=Right
  connections:
  Inv--/RConn1 -- PV--/RConn1 -- C2/RConn1
  C1/RConn1 -- N/RConn1 -- C2/LConn1
  Inv+/RConn1 -- PV+/RConn1 -- C1/LConn1

== system different_inverter_controls_BPS/IBR GFL-SH/IBR/Grid Inverter ==
  note: Harmonic Filter
  Uref : Inport
  10 kvar : spsThreePhaseSeriesRLCLoadLib/Three-Phase Series RLC Load  LConnTagsString=A|B|C  Configuration=Delta  NominalVoltage=Vnom_sec  Vabc=[1e3 1e3 1e3]  Vabcp=[1e3 1e3 1e3]  NominalFrequency=Fnom  UnbalancedPower=off  ActivePower=Pc  InductivePower=0  CapacitivePower=Qc  Pabc=[10e3 9e3 11e3]  QLabc=[100 90 110]  QCabc=[100 90 110]  Pabcp=[10e3 9e3 11e3]  QLabcp=[100 90 110]  QCabcp=[100 90 110]  Measurements=None  LoadType=constant Z
  B1 : spsThreePhaseVIMeasurementLib/Three-Phase V-I Measurement  VoltageMeasurement=phase-to-ground  SetLabelV=off  LabelV=Vabc_B1  Vpu=off  VpuLL=off  CurrentMeasurement=yes  SetLabelI=off  LabelI=Iabc_B1  Ipu=off  Pbase=100e6  Vbase=500e3  OutputType=Magnitude  PhasorSimulation=off  PSBequivalent=0
  Bus Creator : BusCreator  Inputs=2
  Ground : Ground
  L : spsThreePhaseSeriesRLCBranchLib/Three-Phase Series RLC Branch  LConnTagsString=A|B|C  RConnTagsString=A|B|C  BranchType=RL  Resistance=Rchoke*Zbase  Inductance=Lchoke*Zbase/(2*pi*Fnom)  Capacitance=inf  Measurements=None
  Three-Level NPC Converter : spsThreeLevelNPCConverterLib/Three-Level NPC Converter  ModelType=Average model (Uref-controlled)  Ron=1e-3  Rs=1e6  Cs=inf  Vforward=[0,0]  Ron_Diode=1e-3  Rs_Diode=1e6  Cs_Diode=inf  Vf_Diode=1e-3  Rs_CurrentSource=inf  Ron_ACsource=1e-3
  XFR : spsThreePhaseTransformerTwoWindingsLib/Three-Phase Transformer (Two Windings)  Winding1Connection=Delta (D1)  Winding2Connection=Delta (D1)  CoreType=Three single-phase transformers  SetSaturation=off  Hysteresis=off  DataFile='hysteresis'  SetInitialFlux=off  Measurements=None  UNITS=pu  NominalPower=[100e6, f ]  Winding1="[Vnom_prim,  1e-6, 0.0586 ]"  Winding2="[ Vnom_sec,  1e-6, 0.0586 ]"  Rm=500  Lm=500  L0=0.5  Saturation=[ 0,0 ; 0.0024,1.2 ; 1.0,1.52 ]  InitialFluxes=[ 0.8 , -0.8 , 0.7 ]  BreakLoop=off  DiscreteSolver=Trapezoidal iterative  DataType=off  TransfoNumber=1
  A : PMIOPort  Side=Right
  B : PMIOPort  Port=2  Side=Right
  C : PMIOPort  Port=3  Side=Right
  Inv+ : PMIOPort  Port=4  Side=Left
  N : PMIOPort  Port=5  Side=Left
  Inv-- : PMIOPort  Port=6  Side=Left
  m : Outport  VectorParamsAs1DForOutWhenUnconnected=off
  wires:
  B1/1 -> Bus Creator/1  "Vabc"
  B1/2 -> Bus Creator/2  "Iabc"
  Bus Creator/1 -> m/1
  Ground/1 -> Three-Level NPC Converter/2
  Uref/1 -> Three-Level NPC Converter/1
  connections:
  B1/RConn3 -- C/RConn1
  B1/RConn2 -- B/RConn1
  B1/RConn1 -- A/RConn1
  10 kvar/LConn1 -- XFR/RConn1 -- L/RConn1
  L/RConn3 -- XFR/RConn3 -- 10 kvar/LConn3
  L/RConn2 -- XFR/RConn2 -- 10 kvar/LConn2
  XFR/LConn3 -- B1/LConn3
  XFR/LConn2 -- B1/LConn2
  XFR/LConn1 -- B1/LConn1
  Three-Level NPC Converter/RConn3 -- Inv--/RConn1
  Three-Level NPC Converter/LConn2 -- L/LConn2
  N/RConn1 -- Three-Level NPC Converter/RConn2
  Three-Level NPC Converter/RConn1 -- Inv+/RConn1
  Three-Level NPC Converter/LConn3 -- L/LConn3
  Three-Level NPC Converter/LConn1 -- L/LConn1

== system different_inverter_controls_BPS/IBR GFL-SH/IBR/Inverter Control ==
  Vabc_prim : Inport  PortDimensions=3
  Iabc_prim : Inport  Port=2  PortDimensions=3
  Idq_ref : Inport  Port=3
  Current Control : Subsystem  TreatAsAtomicUnit=on
  Demux : Demux  Outputs=2
  From : From  Commented=on  GotoTag=idiqPRef
  Overmodulation : spsOvermodulationLib/Overmodulation  Commented=through  OverModType=Flat top
  Scope : Scope  NumInputPorts=2
  Unit Delay : UnitDelay  SampleTime=Ts_Control  HasFrameUpgradeWarning=on
  Voltage Loop : Subsystem
  current limiter : Subsystem  mask{limMax=clMax, limMin=clMin}
      mask prompts: limMax "Max current limit (pu)"; limMin "Min current limit (pu)"
  Uref : Outport  VectorParamsAs1DForOutWhenUnconnected=off
  wires:
  [IdIqref] -> Current Control/4(IdIq_ref)
  [idiqPRef] -> Scope/2
  [wt] -> Current Control/1(wt)
  Idq_ref/1 -> [IdIqref]
  Voltage Loop/1(wt) -> [wt]
  Demux/2 -> [Vq_meas]
  Demux/1 -> [Vd_meas]
  Vabc_prim/1 -> Voltage Loop/1(Vabc_prim)
  Voltage Loop/3(IdIq_prim) -> [idiqPRef]
  [idiqPRef] -> current limiter/1(idiqPref)
  current limiter/1(idiqPRefL) -> Scope/1, [idiqPRefL]
  Unit Delay/1 -> Overmodulation/1
  Overmodulation/1 -> Uref/1
  Current Control/1(Uabc) -> Unit Delay/1
  Voltage Loop/2(VdVq_prim) -> Demux/1, Current Control/2(VdVq_meas)
  Iabc_prim/1 -> Voltage Loop/2(Iabc_prim)
  [idiqPRefL] -> Current Control/3(IdIq_meas)

== system different_inverter_controls_BPS/IBR GFL-SH/IBR/Measures ==
  Grid : Inport
  IBR : Inport  Port=2
  Bus Creator : BusCreator  Inputs=2
  Bus Creator1 : BusCreator  Inputs=4
  Bus Selector2 : BusSelector  OutputSignals=Vabc,Iabc
  "Power (3ph, Instantaneous)" : spsPower3phInstantaneousLib/Power (3ph, Instantaneous)
  Scope : Scope
  m : Outport  VectorParamsAs1DForOutWhenUnconnected=off
  wires:
  Bus Creator1/1 -> Bus Creator/1  "Grid"
  "Power (3ph, Instantaneous)"/2 -> Bus Creator1/4  "Q"
  Grid/1 -> Bus Selector2/1
  IBR/1 -> Bus Creator/2  "Battery"
  Bus Creator/1 -> m/1
  "Power (3ph, Instantaneous)"/1 -> Scope/1, Bus Creator1/3  "P"
  Bus Selector2/2 -> Bus Creator1/2, "Power (3ph, Instantaneous)"/2  "<Iabc>"
  Bus Selector2/1 -> Bus Creator1/1, "Power (3ph, Instantaneous)"/1  "<Vabc>"

== system different_inverter_controls_BPS/IBR GFL-SH/IBR/Power Control Loop ==
  m_PQ : Inport
  PQref_f : Inport  Port=2
  Compute PQ : Subsystem
  "P,Q Control " : Subsystem  TreatAsAtomicUnit=on
  to PU : Gain  Gain=1/Pnom
  Idq_ref : Outport  VectorParamsAs1DForOutWhenUnconnected=off
  wires:
  to PU/1 -> "P,Q Control "/1(PQref)
  m_PQ/1 -> Compute PQ/1(m)
  Compute PQ/1(PQm) -> "P,Q Control "/2(m)
  "P,Q Control "/1(Idq_ref) -> Idq_ref/1
  PQref_f/1 -> to PU/1

== system different_inverter_controls_BPS/IBR-GFM PV Droop/IBR/ Reference  ==
  Clock : Clock  Commented=on
  Constant1 : Constant  Commented=on  Value=0  SampleTime=Ts_Control
  Constant2 : Constant  Value=110e6*.9  SampleTime=Ts_Control
  Constant3 : Constant  Commented=on  Value=55e6*.9  SampleTime=Ts_Control
  Digital Clock : DigitalClock  Commented=on  SampleTime=Ts_Control
  If : If  Commented=on  IfExpression=u1>=0
  If Action Subsystem : Subsystem  Commented=on  TreatAsAtomicUnit=on
  If Action Subsystem1 : Subsystem  Commented=on  TreatAsAtomicUnit=on
  Merge : Merge  Commented=on
  Mux3 : Mux  Inputs=2
  Pref : Subsystem  Commented=on
  Qref : Subsystem
  Scope : Scope
  tag scope: BESS_PQf_ref=global
  wires:
  Digital Clock/1 -> If/1
  Mux3/1 -> Scope/1, [BESS_PQf_ref]
  If Action Subsystem1/1(Out1) -> Merge/2
  If/2 -> If Action Subsystem1/Action
  Pref/1(Out1) -> If Action Subsystem/1(In1)
  If/1 -> If Action Subsystem/Action
  If Action Subsystem/1(Out1) -> Merge/1
  Constant1/1 -> If Action Subsystem1/1(In1)
  Qref/1(Out1) -> Mux3/2
  Constant2/1 -> Mux3/1

== system different_inverter_controls_BPS/IBR-GFM PV Droop/IBR/DC Link ==
  C1 : spsSeriesRLCBranchLib/Series RLC Branch  LConnTagsString=__new0  RConnTagsString=__new0  BranchType=RC  Resistance=10e-5  Inductance=1.0  SetiL0=off  InitialCurrent=0  Capacitance=inv1.C/2  Setx0=on  InitialVoltage=Vdc/2  Measurements=None
  C2 : spsSeriesRLCBranchLib/Series RLC Branch  LConnTagsString=__new0  RConnTagsString=__new0  BranchType=RC  Resistance=10e-5  Inductance=1.0  SetiL0=off  InitialCurrent=0  Capacitance=inv1.C/2  Setx0=on  InitialVoltage=Vdc/2  Measurements=None
  C3 : spsSeriesRLCBranchLib/Series RLC Branch  Commented=on  LConnTagsString=__new0  RConnTagsString=__new0  BranchType=RC  Resistance=10e-5  Inductance=1.0  SetiL0=off  InitialCurrent=0  Capacitance=Clink  Setx0=on  InitialVoltage=Vnom_dc/2  Measurements=None
  PV+ : PMIOPort  Side=Left
  PV-- : PMIOPort  Port=2  Side=Left
  Inv+ : PMIOPort  Port=3  Side=Right
  N : PMIOPort  Port=4  Side=Right
  Inv-- : PMIOPort  Port=5  Side=Right
  connections:
  C1/LConn1 -- PV+/RConn1 -- Inv+/RConn1
  C2/LConn1 -- N/RConn1 -- C1/RConn1
  C2/RConn1 -- PV--/RConn1 -- Inv--/RConn1

== system different_inverter_controls_BPS/IBR-GFM PV Droop/IBR/Grid Inverter ==
  note: Harmonic Filter
  Uref : Inport
  10 kvar1 : spsThreePhaseSeriesRLCLoadLib/Three-Phase Series RLC Load  Commented=on  LConnTagsString=A|B|C  Configuration=Delta  NominalVoltage=Vpp  Vabc=[1e3 1e3 1e3]  Vabcp=[1e3 1e3 1e3]  NominalFrequency=f  UnbalancedPower=off  ActivePower=Pc  InductivePower=0  CapacitivePower=Qc  Pabc=[10e3 9e3 11e3]  QLabc=[100 90 110]  QCabc=[100 90 110]  Pabcp=[10e3 9e3 11e3]  QLabcp=[100 90 110]  QCabcp=[100 90 110]  Measurements=None  LoadType=constant Z
  10 kvar2 : spsThreePhaseSeriesRLCLoadLib/Three-Phase Series RLC Load  Commented=on  LConnTagsString=A|B|C  Configuration=Delta  NominalVoltage=Vpp  Vabc=[1e3 1e3 1e3]  Vabcp=[1e3 1e3 1e3]  NominalFrequency=f  UnbalancedPower=off  ActivePower=Pc  InductivePower=0  CapacitivePower=Qc  Pabc=[10e3 9e3 11e3]  QLabc=[100 90 110]  QCabc=[100 90 110]  Pabcp=[10e3 9e3 11e3]  QLabcp=[100 90 110]  QCabcp=[100 90 110]  Measurements=None  LoadType=constant Z
  B1 : spsThreePhaseVIMeasurementLib/Three-Phase V-I Measurement  VoltageMeasurement=phase-to-ground  SetLabelV=off  LabelV=Vabc_B1  Vpu=off  VpuLL=off  CurrentMeasurement=yes  SetLabelI=off  LabelI=Iabc_B1  Ipu=off  Pbase=100e6  Vbase=500e3  OutputType=Magnitude  PhasorSimulation=off  PSBequivalent=0
  B2 : spsThreePhaseVIMeasurementLib/Three-Phase V-I Measurement  Commented=on  VoltageMeasurement=no  SetLabelV=off  LabelV=Vabc_B1  Vpu=off  VpuLL=off  CurrentMeasurement=yes  SetLabelI=off  LabelI=Iabc_B1  Ipu=on  Pbase=50e6  Vbase=Vnom_sec  OutputType=Magnitude  PhasorSimulation=off  PSBequivalent=0
  B3 : spsThreePhaseVIMeasurementLib/Three-Phase V-I Measurement  VoltageMeasurement=phase-to-ground  SetLabelV=on  LabelV=Vinv  Vpu=on  VpuLL=off  CurrentMeasurement=yes  SetLabelI=on  LabelI=Iinv  Ipu=on  Pbase=110e6  Vbase=Vpp  OutputType=Magnitude  PhasorSimulation=off  PSBequivalent=0
  B4 : spsThreePhaseVIMeasurementLib/Three-Phase V-I Measurement  Commented=on  VoltageMeasurement=phase-to-ground  SetLabelV=on  LabelV=Vinv  Vpu=on  VpuLL=off  CurrentMeasurement=yes  SetLabelI=on  LabelI=Igrid  Ipu=on  Pbase=55e6  Vbase=Vpp  OutputType=Magnitude  PhasorSimulation=off  PSBequivalent=0
  Bus Creator : BusCreator  Inputs=2
  Cf : spsThreePhaseSeriesRLCBranchLib/Three-Phase Series RLC Branch  LConnTagsString=A|B|C  RConnTagsString=A|B|C  BranchType=RC  Resistance=inv1.Rf  Inductance=inv1.L  Capacitance=inv1.Cf  Measurements=None
  Ground : Ground
  Ground1 : spsGroundLib/Ground  LConnTagsString=a
  L1 : spsThreePhaseSeriesRLCBranchLib/Three-Phase Series RLC Branch  LConnTagsString=A|B|C  RConnTagsString=A|B|C  BranchType=RL  Resistance=Rchoke*Zbase  Inductance=inv1.L  Capacitance=inf  Measurements=None
  L2 : spsThreePhaseSeriesRLCBranchLib/Three-Phase Series RLC Branch  Commented=on  LConnTagsString=A|B|C  RConnTagsString=A|B|C  BranchType=RL  Resistance=Rchoke*Zbase  Inductance=Lchoke*Zbase/(2*pi*Fnom)  Capacitance=inf  Measurements=None
  L3 : spsThreePhaseSeriesRLCBranchLib/Three-Phase Series RLC Branch  Commented=on  LConnTagsString=A|B|C  RConnTagsString=A|B|C  BranchType=RL  Resistance=inv1.R  Inductance=inv1.L  Capacitance=inf  Measurements=None
  "Power (3ph, Instantaneous)" : spsPower3phInstantaneousLib/Power (3ph, Instantaneous)
  Scope : Scope  NumInputPorts=2
  Scope1 : Scope  NumInputPorts=2
  Scope2 : Scope
  Three-Level NPC Converter : spsThreeLevelNPCConverterLib/Three-Level NPC Converter  ModelType=Average model (Uref-controlled)  Ron=1e-3  Rs=1e6  Cs=inf  Vforward=[0,0]  Ron_Diode=1e-3  Rs_Diode=1e6  Cs_Diode=inf  Vf_Diode=1e-3  Rs_CurrentSource=inf  Ron_ACsource=1e-3
  XFR : spsThreePhaseTransformerTwoWindingsLib/Three-Phase Transformer (Two Windings)  Winding1Connection=Yg  Winding2Connection=Yg  CoreType=Three single-phase transformers  SetSaturation=off  Hysteresis=off  DataFile='hysteresis'  SetInitialFlux=off  Measurements=None  UNITS=pu  NominalPower=[200e6, f ]  Winding1="[Vpp,  1e-6, 0.0586  ]"  Winding2="[ Vnom_prim,  1e-6, 0.0586  ]"  Rm=500  Lm=500  L0=0.5  Saturation=[ 0,0 ; 0.0024,1.2 ; 1.0,1.52 ]  InitialFluxes=[ 0.8 , -0.8 , 0.7 ]  BreakLoop=off  DiscreteSolver=Trapezoidal iterative  DataType=off  TransfoNumber=1
  XFR1 : spsThreePhaseTransformerTwoWindingsLib/Three-Phase Transformer (Two Windings)  Commented=on  Winding1Connection=Delta (D1)  Winding2Connection=Delta (D1)  CoreType=Three single-phase transformers  SetSaturation=off  Hysteresis=off  DataFile='hysteresis'  SetInitialFlux=off  Measurements=None  UNITS=pu  NominalPower=[100e6, f ]  Winding1="[Vnom_prim,  1e-6, 0.0586 ]"  Winding2="[ Vnom_sec,  1e-6, 0.0586 ]"  Rm=500  Lm=500  L0=0.5  Saturation=[ 0,0 ; 0.0024,1.2 ; 1.0,1.52 ]  InitialFluxes=[ 0.8 , -0.8 , 0.7 ]  BreakLoop=off  DiscreteSolver=Trapezoidal iterative  DataType=off  TransfoNumber=1
  Inv+ : PMIOPort  Side=Left
  N : PMIOPort  Port=2  Side=Left
  Inv-- : PMIOPort  Port=3  Side=Left
  A : PMIOPort  Port=4  Side=Right
  B : PMIOPort  Port=5  Side=Right
  C : PMIOPort  Port=6  Side=Right
  m : Outport  VectorParamsAs1DForOutWhenUnconnected=off
  tag scope: ICabc=global
  wires:
  Ground/1 -> Three-Level NPC Converter/2
  Bus Creator/1 -> m/1
  B1/2 -> "Power (3ph, Instantaneous)"/2, Scope1/1, Bus Creator/2, [ICabc]  "Iabc"
  B1/1 -> Bus Creator/1, "Power (3ph, Instantaneous)"/1, Scope/1  "Vabc"
  Uref/1 -> Three-Level NPC Converter/1
  [Vinv] -> Scope/2
  [Iinv] -> Scope1/2
  "Power (3ph, Instantaneous)"/1 -> Scope2/1
  connections:
  N/RConn1 -- Three-Level NPC Converter/RConn2
  Three-Level NPC Converter/RConn3 -- Inv--/RConn1
  Three-Level NPC Converter/RConn1 -- Inv+/RConn1
  Three-Level NPC Converter/LConn2 -- L1/LConn2
  Three-Level NPC Converter/LConn1 -- L1/LConn1
  Three-Level NPC Converter/LConn3 -- L1/LConn3
  L2/RConn2 -- 10 kvar2/LConn2
  L2/RConn3 -- 10 kvar2/LConn3
  10 kvar2/LConn1 -- L2/RConn1
  Ground1/LConn1 -- Cf/RConn1 -- Cf/RConn3 -- Cf/RConn2
  B1/LConn1 -- L1/RConn1
  B1/LConn2 -- L1/RConn2
  B1/LConn3 -- L1/RConn3
  B1/RConn1 -- 10 kvar1/LConn1 -- Cf/LConn1 -- B3/LConn1
  B1/RConn2 -- Cf/LConn2 -- B3/LConn2 -- 10 kvar1/LConn2
  B1/RConn3 -- 10 kvar1/LConn3 -- Cf/LConn3 -- B3/LConn3
  XFR/LConn1 -- B3/RConn1
  B3/RConn2 -- XFR/LConn2
  B3/RConn3 -- XFR/LConn3
  XFR/RConn1 -- A/RConn1
  XFR/RConn2 -- B/RConn1
  XFR/RConn3 -- C/RConn1

== system different_inverter_controls_BPS/IBR-GFM PV Droop/IBR/Inverter Control ==
  Vabc_prim : Inport  PortDimensions=3
  Iabc_prim : Inport  Port=2  PortDimensions=3
  theta : Inport  Port=3
  Vdref : Inport  Port=4
  V_inv_mag : Inport  Port=5
  " voltage control " : Subsystem
  Conversions : Subsystem
  Current Control : Subsystem  TreatAsAtomicUnit=on
  Demux : Demux  Outputs=2
  From : From  Commented=on  GotoTag=Iabc_B5  TagVisibility=global
  From10 : From  Commented=on  GotoTag=idiqPRefL
  From5 : From  Commented=on  GotoTag=theta  TagVisibility=global
  From7 : From  Commented=on  GotoTag=idiqPRef
  Goto5 : Goto  Commented=on  GotoTag=Vabc_prim
  Overmodulation : spsOvermodulationLib/Overmodulation  Commented=on  OverModType=Flat top
  Scope : Scope  NumInputPorts=2
  Scope1 : Scope
  Scope2 : Scope
  Unit Delay : UnitDelay  SampleTime=Ts_Control  HasFrameUpgradeWarning=on
  current limiter : Subsystem  mask{limMax=clMax, limMin=clMin}
      mask prompts: limMax "Max current limit (pu)"; limMin "Min current limit (pu)"
  Uref : Outport  VectorParamsAs1DForOutWhenUnconnected=off
  tag scope: Vd_meas=global, Vq_meas=global, idiqgrid=global, theta=global
  wires:
  " voltage control "/1(IdIq_ref.) -> Scope2/1, [IdIqref]
  [Vq_meas] -> " voltage control "/2(Vq)
  Iabc_prim/1 -> Conversions/2(Iabc_prim)
  Conversions/2(VdVq_prim) -> Current Control/2(VdVq_meas), Scope1/1, Demux/1
  Current Control/1(Uabc) -> Unit Delay/1
  Conversions/3(IdIq_prim) -> [idiqPRef]
  [idiqPRef] -> Current Control/3(IdIq_meas)
  Vabc_prim/1 -> Conversions/1(Vabc_prim), Goto5/1
  Conversions/1(wt) -> [wt_GFL]
  theta/1 -> [theta]
  [Vd_meas] -> " voltage control "/1(Vd_meas)
  Demux/1 -> [Vd_meas]
  Demux/2 -> [Vq_meas]
  [idiqPRef] -> Scope/2
  current limiter/1(idiqPRefL) -> Scope/1, [idiqPRefL]
  Vdref/1 -> " voltage control "/3(Vdref)
  [IdIqref] -> current limiter/1(idiqPref)
  [IdIqref] -> Current Control/4(IdIq_ref)
  V_inv_mag/1 -> current limiter/2(V_inv_mag)
  Conversions/4(IdIq_grid) -> [idiqgrid]
  From/1 -> Conversions/3(Iabc_grid)
  [theta] -> Current Control/1(wt)
  Unit Delay/1 -> Uref/1

== system different_inverter_controls_BPS/IBR-GFM PV Droop/IBR/Measures ==
  Grid : Inport
  Battery : Inport  Port=2
  Bus Creator : BusCreator  Inputs=2
  Bus Creator1 : BusCreator  Inputs=4
  Bus Selector2 : BusSelector  OutputSignals=Vabc,Iabc
  "Power (3ph, Instantaneous)" : spsPower3phInstantaneousLib/Power (3ph, Instantaneous)
  Scope : Scope
  m : Outport  VectorParamsAs1DForOutWhenUnconnected=off
  wires:
  Bus Selector2/1 -> "Power (3ph, Instantaneous)"/1, Bus Creator1/1  "<Vabc>"
  Bus Selector2/2 -> "Power (3ph, Instantaneous)"/2, Bus Creator1/2  "<Iabc>"
  "Power (3ph, Instantaneous)"/1 -> Bus Creator1/3, Scope/1  "P"
  Bus Creator/1 -> m/1
  Battery/1 -> Bus Creator/2  "Battery"
  Grid/1 -> Bus Selector2/1
  "Power (3ph, Instantaneous)"/2 -> Bus Creator1/4  "Q"
  Bus Creator1/1 -> Bus Creator/1  "Grid"

== system different_inverter_controls_BPS/IBR-GFM PV Droop/IBR/Power Controller ==
  m_PQ : Inport
  PQref_f : Inport  Port=2
  Input : Inport  Port=3
  fsys : Inport  Port=4
  V_inv_mag : Inport  Port=5
  -180 < alpha < 180 : spsPMUPLLBasedPositiveSequenceLib/PMU (PLL-Based, Positive-Sequence)/-180 < alpha < 180  Commented=on  SystemSampleTime=-1  VariantActivationTime=update diagram  AllowFlexibleInterface=on  Latency=0  AutoFrameSizeCalculation=off
  Compute PQ : Subsystem
  Goto4 : Goto  Commented=on  GotoTag=theta_inv  TagVisibility=global
  "P,Q Control " : Subsystem  TreatAsAtomicUnit=on
  Scope : Scope
  Scope1 : Scope
  to PU : Gain  Gain=1/Pnom
  theta : Outport  VectorParamsAs1DForOutWhenUnconnected=off
  Vdref : Outport  Port=2
  wires:
  fsys/1 -> "P,Q Control "/4(fsys)
  Input/1 -> "P,Q Control "/3(w0)
  PQref_f/1 -> to PU/1
  m_PQ/1 -> Compute PQ/1(m)
  to PU/1 -> Scope1/1, "P,Q Control "/1(PQref)
  Compute PQ/1(PQm) -> "P,Q Control "/2(m)
  "P,Q Control "/1(theta) -> theta/1, Goto4/1, Scope/1
  "P,Q Control "/2(Vdref) -> Vdref/1
  V_inv_mag/1 -> "P,Q Control "/5(V_inv_mag)

== system different_inverter_controls_BPS/IBR-GFM Synchro-inverter/Inverter/ Reference  ==
  Constant2 : Constant  Value=110e6*.9  SampleTime=Ts_Control
  Mux3 : Mux  Inputs=2
  Qref : Subsystem
  Scope : Scope
  tag scope: BESS_PQf_ref=global
  wires:
  Constant2/1 -> Mux3/1
  Qref/1(Out1) -> Mux3/2
  Mux3/1 -> [BESS_PQf_ref], Scope/1

== system different_inverter_controls_BPS/IBR-GFM Synchro-inverter/Inverter/DC Link ==
  C1 : spsSeriesRLCBranchLib/Series RLC Branch  LConnTagsString=__new0  RConnTagsString=__new0  BranchType=RC  Resistance=10e-5  Inductance=1.0  SetiL0=off  InitialCurrent=0  Capacitance=inv1.C/2  Setx0=on  InitialVoltage=Vdc/2  Measurements=None
  C2 : spsSeriesRLCBranchLib/Series RLC Branch  LConnTagsString=__new0  RConnTagsString=__new0  BranchType=RC  Resistance=10e-5  Inductance=1.0  SetiL0=off  InitialCurrent=0  Capacitance=inv1.C/2  Setx0=on  InitialVoltage=Vdc/2  Measurements=None
  C3 : spsSeriesRLCBranchLib/Series RLC Branch  Commented=on  LConnTagsString=__new0  RConnTagsString=__new0  BranchType=RC  Resistance=10e-5  Inductance=1.0  SetiL0=off  InitialCurrent=0  Capacitance=Clink  Setx0=on  InitialVoltage=Vnom_dc/2  Measurements=None
  PV+ : PMIOPort  Side=Left
  PV-- : PMIOPort  Port=2  Side=Left
  Inv+ : PMIOPort  Port=3  Side=Right
  N : PMIOPort  Port=4  Side=Right
  Inv-- : PMIOPort  Port=5  Side=Right
  connections:
  Inv--/RConn1 -- PV--/RConn1 -- C2/RConn1
  C1/RConn1 -- N/RConn1 -- C2/LConn1
  Inv+/RConn1 -- PV+/RConn1 -- C1/LConn1
